simulink model "c00005M_harness"  (R2018a)
settings: Solver=FixedStepAuto  StartTime=0.0  StopTime=300  FixedStep=0.1  RelTol=1e-3
undefined symbols (not defined in the file): A1, hmax, PriorityTank, R1, R2, sigbuilder_block, TempThreshold
(part 44 of 50)

== system c00005M_harness/M203/Tank1/Control/Maintenance ==
  Type : Inport
  StartMaintenance : Inport  Port=2
  LiquidLevel : Inport  Port=3
  Chart : Stateflow chart  TreatAsAtomicUnit=on
  LiquidIn : Outport
  LiquidOut : Outport  Port=2
  wires:
  StartMaintenance/1 -> Chart/2(StartMaintenance)
  Type/1 -> Chart/1(Type)
  LiquidLevel/1 -> Chart/3(LiquidLevel)
  Chart/1(LiquidIn) -> LiquidIn/1
  Chart/2(LiquidOut) -> LiquidOut/1

== system c00005M_harness/M203/Tank1/Control/ManualControlLiquidInOut ==
  Fill : Inport
  Empty : Inport  Port=2
  LiquidLevel : Inport  Port=3
  Constant : Constant  Value=hmax*0.9
  Constant1 : Constant  Value=0.001
  Logical Operator{,1..2,4} (4 alike) : Logic  AllPortsSameDT=off  OutDataTypeStr=boolean
  Logical Operator3 : Logic  Operator=NOT  AllPortsSameDT=off  OutDataTypeStr=boolean
  Logical Operator5 : Logic  Operator=NOT  AllPortsSameDT=off  OutDataTypeStr=boolean
  Relational Operator1 : RelationalOperator  Operator=<  OutDataTypeStr=boolean  RndMeth=Simplest
  Relational Operator2 : RelationalOperator  Operator=<  OutDataTypeStr=boolean  RndMeth=Simplest
  LiquidIn : Outport
  LiquidOut : Outport  Port=2
  wires:
  Empty/1 -> Logical Operator1/2
  Constant/1 -> Relational Operator1/2
  Relational Operator1/1 -> Logical Operator/2
  Fill/1 -> Logical Operator/1
  Logical Operator/1 -> Logical Operator5/1, Logical Operator2/1
  Relational Operator2/1 -> Logical Operator1/1
  Logical Operator1/1 -> Logical Operator3/1, Logical Operator4/2
  Constant1/1 -> Relational Operator2/1
  LiquidLevel/1 -> Relational Operator2/2, Relational Operator1/1
  Logical Operator3/1 -> Logical Operator2/2
  Logical Operator2/1 -> LiquidIn/1
  Logical Operator5/1 -> Logical Operator4/1
  Logical Operator4/1 -> LiquidOut/1

== system c00005M_harness/M203/Tank3/Control/Maintenance ==
  Type : Inport
  StartMaintenance : Inport  Port=2
  LiquidLevel : Inport  Port=3
  Chart : Stateflow chart  TreatAsAtomicUnit=on
  LiquidIn : Outport
  LiquidOut : Outport  Port=2
  wires:
  StartMaintenance/1 -> Chart/2(StartMaintenance)
  Type/1 -> Chart/1(Type)
  LiquidLevel/1 -> Chart/3(LiquidLevel)
  Chart/1(LiquidIn) -> LiquidIn/1
  Chart/2(LiquidOut) -> LiquidOut/1

== system c00005M_harness/M203/Tank3/Control/ManualControlLiquidInOut ==
  Fill : Inport
  Empty : Inport  Port=2
  LiquidLevel : Inport  Port=3
  Constant : Constant  Value=hmax*0.9
  Constant1 : Constant  Value=0.001
  Logical Operator : Logic  AllPortsSameDT=off  OutDataTypeStr=boolean
  Logical Operator1 : Logic  Operator=OR  AllPortsSameDT=off  OutDataTypeStr=boolean
  Logical Operator2 : Logic  AllPortsSameDT=off  OutDataTypeStr=boolean
  Logical Operator3 : Logic  Operator=NOT  AllPortsSameDT=off  OutDataTypeStr=boolean
  Logical Operator4 : Logic  AllPortsSameDT=off  OutDataTypeStr=boolean
  Logical Operator5 : Logic  Operator=NOT  AllPortsSameDT=off  OutDataTypeStr=boolean
  Relational Operator1 : RelationalOperator  Operator=<  OutDataTypeStr=boolean  RndMeth=Simplest
  Relational Operator2 : RelationalOperator  Operator=<  OutDataTypeStr=boolean  RndMeth=Simplest
  LiquidIn : Outport
  LiquidOut : Outport  Port=2
  wires:
  Empty/1 -> Logical Operator1/2
  Constant/1 -> Relational Operator1/2
  Relational Operator1/1 -> Logical Operator/2
  Fill/1 -> Logical Operator/1
  Logical Operator/1 -> Logical Operator5/1, Logical Operator2/1
  Relational Operator2/1 -> Logical Operator1/1
  Logical Operator1/1 -> Logical Operator3/1, Logical Operator4/2
  Constant1/1 -> Relational Operator2/1
  LiquidLevel/1 -> Relational Operator2/2, Relational Operator1/1
  Logical Operator3/1 -> Logical Operator2/2
  Logical Operator2/1 -> LiquidIn/1
  Logical Operator5/1 -> Logical Operator4/1
  Logical Operator4/1 -> LiquidOut/1

== system c00005M_harness/M204/Tank1/Control/Maintenance ==
  Type : Inport
  StartMaintenance : Inport  Port=2
  LiquidLevel : Inport  Port=3
  Chart : Stateflow chart  TreatAsAtomicUnit=on
  LiquidIn : Outport
  LiquidOut : Outport  Port=2
  wires:
  StartMaintenance/1 -> Chart/2(StartMaintenance)
  Type/1 -> Chart/1(Type)
  LiquidLevel/1 -> Chart/3(LiquidLevel)
  Chart/1(LiquidIn) -> LiquidIn/1
  Chart/2(LiquidOut) -> LiquidOut/1

== system c00005M_harness/M204/Tank1/Control/ManualControlLiquidInOut ==
  Fill : Inport
  Empty : Inport  Port=2
  LiquidLevel : Inport  Port=3
  Constant : Constant  Value=hmax*0.9
  Constant1 : Constant  Value=0.001
  Logical Operator{,1..2,4} (4 alike) : Logic  AllPortsSameDT=off  OutDataTypeStr=boolean
  Logical Operator3 : Logic  Operator=NOT  AllPortsSameDT=off  OutDataTypeStr=boolean
  Logical Operator5 : Logic  Operator=NOT  AllPortsSameDT=off  OutDataTypeStr=boolean
  Relational Operator1 : RelationalOperator  Operator=<  OutDataTypeStr=boolean  RndMeth=Simplest
  Relational Operator2 : RelationalOperator  Operator=<  OutDataTypeStr=boolean  RndMeth=Simplest
  LiquidIn : Outport
  LiquidOut : Outport  Port=2
  wires:
  Empty/1 -> Logical Operator1/2
  Constant/1 -> Relational Operator1/2
  Relational Operator1/1 -> Logical Operator/2
  Fill/1 -> Logical Operator/1
  Logical Operator/1 -> Logical Operator5/1, Logical Operator2/1
  Relational Operator2/1 -> Logical Operator1/1
  Logical Operator1/1 -> Logical Operator3/1, Logical Operator4/2
  Constant1/1 -> Relational Operator2/1
  LiquidLevel/1 -> Relational Operator2/2, Relational Operator1/1
  Logical Operator3/1 -> Logical Operator2/2
  Logical Operator2/1 -> LiquidIn/1
  Logical Operator5/1 -> Logical Operator4/1
  Logical Operator4/1 -> LiquidOut/1

== system c00005M_harness/M204/Tank3/Control/Maintenance ==
  Type : Inport
  StartMaintenance : Inport  Port=2
  LiquidLevel : Inport  Port=3
  Chart : Stateflow chart  TreatAsAtomicUnit=on
  LiquidIn : Outport
  LiquidOut : Outport  Port=2
  wires:
  StartMaintenance/1 -> Chart/2(StartMaintenance)
  Type/1 -> Chart/1(Type)
  LiquidLevel/1 -> Chart/3(LiquidLevel)
  Chart/1(LiquidIn) -> LiquidIn/1
  Chart/2(LiquidOut) -> LiquidOut/1

== system c00005M_harness/M204/Tank3/Control/ManualControlLiquidInOut ==
  Fill : Inport
  Empty : Inport  Port=2
  LiquidLevel : Inport  Port=3
  Constant : Constant  Value=hmax*0.9
  Constant1 : Constant  Value=0.001
  Logical Operator : Logic  AllPortsSameDT=off  OutDataTypeStr=boolean
  Logical Operator1 : Logic  AllPortsSameDT=off  OutDataTypeStr=boolean
  Logical Operator2 : Logic  Operator=OR  AllPortsSameDT=off  OutDataTypeStr=boolean
  Logical Operator3 : Logic  Operator=NOT  AllPortsSameDT=off  OutDataTypeStr=boolean
  Logical Operator4 : Logic  AllPortsSameDT=off  OutDataTypeStr=boolean
  Logical Operator5 : Logic  Operator=NOT  AllPortsSameDT=off  OutDataTypeStr=boolean
  Relational Operator1 : RelationalOperator  Operator=<  OutDataTypeStr=boolean  RndMeth=Simplest
  Relational Operator2 : RelationalOperator  Operator=<  OutDataTypeStr=boolean  RndMeth=Simplest
  LiquidIn : Outport
  LiquidOut : Outport  Port=2
  wires:
  Empty/1 -> Logical Operator1/2
  Constant/1 -> Relational Operator1/2
  Relational Operator1/1 -> Logical Operator/2
  Fill/1 -> Logical Operator/1
  Logical Operator/1 -> Logical Operator5/1, Logical Operator2/1
  Relational Operator2/1 -> Logical Operator1/1
  Logical Operator1/1 -> Logical Operator3/1, Logical Operator4/2
  Constant1/1 -> Relational Operator2/1
  LiquidLevel/1 -> Relational Operator2/2, Relational Operator1/1
  Logical Operator3/1 -> Logical Operator2/2
  Logical Operator2/1 -> LiquidIn/1
  Logical Operator5/1 -> Logical Operator4/1
  Logical Operator4/1 -> LiquidOut/1

== system c00005M_harness/M205/Tank1/Control/Maintenance ==
  Type : Inport
  StartMaintenance : Inport  Port=2
  LiquidLevel : Inport  Port=3
  Chart : Stateflow chart  TreatAsAtomicUnit=on
  LiquidIn : Outport
  LiquidOut : Outport  Port=2
  wires:
  StartMaintenance/1 -> Chart/2(StartMaintenance)
  Type/1 -> Chart/1(Type)
  LiquidLevel/1 -> Chart/3(LiquidLevel)
  Chart/1(LiquidIn) -> LiquidIn/1
  Chart/2(LiquidOut) -> LiquidOut/1

== system c00005M_harness/M205/Tank1/Control/ManualControlLiquidInOut ==
  Fill : Inport
  Empty : Inport  Port=2
  LiquidLevel : Inport  Port=3
  Constant : Constant  Value=hmax*0.9
  Constant1 : Constant  Value=0.001
  Logical Operator{,1..2,4} (4 alike) : Logic  AllPortsSameDT=off  OutDataTypeStr=boolean
  Logical Operator3 : Logic  Operator=NOT  AllPortsSameDT=off  OutDataTypeStr=boolean
  Logical Operator5 : Logic  Operator=NOT  AllPortsSameDT=off  OutDataTypeStr=boolean
  Relational Operator1 : RelationalOperator  Operator=<  OutDataTypeStr=boolean  RndMeth=Simplest
  Relational Operator2 : RelationalOperator  Operator=<  OutDataTypeStr=boolean  RndMeth=Simplest
  LiquidIn : Outport
  LiquidOut : Outport  Port=2
  wires:
  Empty/1 -> Logical Operator1/2
  Constant/1 -> Relational Operator1/2
  Relational Operator1/1 -> Logical Operator/2
  Fill/1 -> Logical Operator/1
  Logical Operator/1 -> Logical Operator5/1, Logical Operator2/1
  Relational Operator2/1 -> Logical Operator1/1
  Logical Operator1/1 -> Logical Operator3/1, Logical Operator4/2
  Constant1/1 -> Relational Operator2/1
  LiquidLevel/1 -> Relational Operator2/2, Relational Operator1/1
  Logical Operator3/1 -> Logical Operator2/2
  Logical Operator2/1 -> LiquidIn/1
  Logical Operator5/1 -> Logical Operator4/1
  Logical Operator4/1 -> LiquidOut/1

== system c00005M_harness/M205/Tank3/Control/Maintenance ==
  Type : Inport
  StartMaintenance : Inport  Port=2
  LiquidLevel : Inport  Port=3
  Chart : Stateflow chart  TreatAsAtomicUnit=on
  LiquidIn : Outport
  LiquidOut : Outport  Port=2
  wires:
  StartMaintenance/1 -> Chart/2(StartMaintenance)
  Type/1 -> Chart/1(Type)
  LiquidLevel/1 -> Chart/3(LiquidLevel)
  Chart/1(LiquidIn) -> LiquidIn/1
  Chart/2(LiquidOut) -> LiquidOut/1

== system c00005M_harness/M205/Tank3/Control/ManualControlLiquidInOut ==
  Fill : Inport
  Empty : Inport  Port=2
  LiquidLevel : Inport  Port=3
  Constant : Constant  Value=hmax*0.9
  Constant1 : Constant  Value=0.001
  Logical Operator{,1..2,4} (4 alike) : Logic  AllPortsSameDT=off  OutDataTypeStr=boolean
  Logical Operator5 : Logic  Operator=NOT  AllPortsSameDT=off  OutDataTypeStr=boolean
  Relational Operator1 : RelationalOperator  Operator=<  OutDataTypeStr=boolean  RndMeth=Simplest
  Relational Operator2 : RelationalOperator  Operator=<  OutDataTypeStr=boolean  RndMeth=Simplest
  LiquidIn : Outport
  LiquidOut : Outport  Port=2
  wires:
  Empty/1 -> Logical Operator1/2
  Constant/1 -> Relational Operator1/2
  Relational Operator1/1 -> Logical Operator/2
  Fill/1 -> Logical Operator/1
  Logical Operator/1 -> Logical Operator5/1, Logical Operator2/1
  Relational Operator2/1 -> Logical Operator1/1
  Constant1/1 -> Relational Operator2/1
  LiquidLevel/1 -> Relational Operator2/2, Relational Operator1/1
  Logical Operator1/1 -> Logical Operator2/2, Logical Operator4/2
  Logical Operator2/1 -> LiquidIn/1
  Logical Operator5/1 -> Logical Operator4/1
  Logical Operator4/1 -> LiquidOut/1

== system c00005M_harness/M206/Tank1/Control/Maintenance ==
  Type : Inport
  StartMaintenance : Inport  Port=2
  LiquidLevel : Inport  Port=3
  Chart : Stateflow chart  TreatAsAtomicUnit=on
  LiquidIn : Outport
  LiquidOut : Outport  Port=2
  wires:
  StartMaintenance/1 -> Chart/2(StartMaintenance)
  Type/1 -> Chart/1(Type)
  LiquidLevel/1 -> Chart/3(LiquidLevel)
  Chart/1(LiquidIn) -> LiquidIn/1
  Chart/2(LiquidOut) -> LiquidOut/1

== system c00005M_harness/M206/Tank1/Control/ManualControlLiquidInOut ==
  Fill : Inport
  Empty : Inport  Port=2
  LiquidLevel : Inport  Port=3
  Constant : Constant  Value=hmax*0.9
  Constant1 : Constant  Value=0.001
  Logical Operator{,1..2,4} (4 alike) : Logic  AllPortsSameDT=off  OutDataTypeStr=boolean
  Logical Operator3 : Logic  Operator=NOT  AllPortsSameDT=off  OutDataTypeStr=boolean
  Logical Operator5 : Logic  Operator=NOT  AllPortsSameDT=off  OutDataTypeStr=boolean
  Relational Operator1 : RelationalOperator  Operator=<  OutDataTypeStr=boolean  RndMeth=Simplest
  Relational Operator2 : RelationalOperator  Operator=<  OutDataTypeStr=boolean  RndMeth=Simplest
  LiquidIn : Outport
  LiquidOut : Outport  Port=2
  wires:
  Empty/1 -> Logical Operator1/2
  Constant/1 -> Relational Operator1/2
  Relational Operator1/1 -> Logical Operator/2
  Fill/1 -> Logical Operator/1
  Logical Operator/1 -> Logical Operator5/1, Logical Operator2/1
  Relational Operator2/1 -> Logical Operator1/1
  Logical Operator1/1 -> Logical Operator3/1, Logical Operator4/2
  Constant1/1 -> Relational Operator2/1
  LiquidLevel/1 -> Relational Operator2/2, Relational Operator1/1
  Logical Operator3/1 -> Logical Operator2/2
  Logical Operator2/1 -> LiquidIn/1
  Logical Operator5/1 -> Logical Operator4/1
  Logical Operator4/1 -> LiquidOut/1

== system c00005M_harness/M206/Tank3/Control/Maintenance ==
  Type : Inport
  StartMaintenance : Inport  Port=2
  LiquidLevel : Inport  Port=3
  Chart : Stateflow chart  TreatAsAtomicUnit=on
  LiquidIn : Outport
  LiquidOut : Outport  Port=2
  wires:
  StartMaintenance/1 -> Chart/2(StartMaintenance)
  Type/1 -> Chart/1(Type)
  LiquidLevel/1 -> Chart/3(LiquidLevel)
  Chart/1(LiquidIn) -> LiquidIn/1
  Chart/2(LiquidOut) -> LiquidOut/1

== system c00005M_harness/M206/Tank3/Control/ManualControlLiquidInOut ==
  Fill : Inport
  Empty : Inport  Port=2
  LiquidLevel : Inport  Port=3
  Constant : Constant  Value=hmax*0.9
  Constant1 : Constant  Value=0.001
  Logical Operator : Logic  AllPortsSameDT=off  OutDataTypeStr=boolean
  Logical Operator1 : Logic  AllPortsSameDT=off  OutDataTypeStr=boolean
  Logical Operator2 : Logic  AllPortsSameDT=off  OutDataTypeStr=boolean
  Logical Operator3 : Logic  Operator=NOT  AllPortsSameDT=off  OutDataTypeStr=boolean
  Logical Operator4 : Logic  Operator=OR  AllPortsSameDT=off  OutDataTypeStr=boolean
  Logical Operator5 : Logic  Operator=NOT  AllPortsSameDT=off  OutDataTypeStr=boolean
  Relational Operator1 : RelationalOperator  Operator=<  OutDataTypeStr=boolean  RndMeth=Simplest
  Relational Operator2 : RelationalOperator  Operator=<  OutDataTypeStr=boolean  RndMeth=Simplest
  LiquidIn : Outport
  LiquidOut : Outport  Port=2
  wires:
  Empty/1 -> Logical Operator1/2
  Constant/1 -> Relational Operator1/2
  Relational Operator1/1 -> Logical Operator/2
  Fill/1 -> Logical Operator/1
  Logical Operator/1 -> Logical Operator5/1, Logical Operator2/1
  Relational Operator2/1 -> Logical Operator1/1
  Logical Operator1/1 -> Logical Operator3/1, Logical Operator4/2
  Constant1/1 -> Relational Operator2/1
  LiquidLevel/1 -> Relational Operator2/2, Relational Operator1/1
  Logical Operator3/1 -> Logical Operator2/2
  Logical Operator2/1 -> LiquidIn/1
  Logical Operator5/1 -> Logical Operator4/1
  Logical Operator4/1 -> LiquidOut/1

== system c00005M_harness/M207/Tank1/Control/Maintenance ==
  Type : Inport
  StartMaintenance : Inport  Port=2
  LiquidLevel : Inport  Port=3
  Chart : Stateflow chart  TreatAsAtomicUnit=on
  LiquidIn : Outport
  LiquidOut : Outport  Port=2
  wires:
  StartMaintenance/1 -> Chart/2(StartMaintenance)
  Type/1 -> Chart/1(Type)
  LiquidLevel/1 -> Chart/3(LiquidLevel)
  Chart/1(LiquidIn) -> LiquidIn/1
  Chart/2(LiquidOut) -> LiquidOut/1

== system c00005M_harness/M207/Tank1/Control/ManualControlLiquidInOut ==
  Fill : Inport
  Empty : Inport  Port=2
  LiquidLevel : Inport  Port=3
  Constant : Constant  Value=hmax*0.9
  Constant1 : Constant  Value=0.001
  Logical Operator{,1..2,4} (4 alike) : Logic  AllPortsSameDT=off  OutDataTypeStr=boolean
  Logical Operator3 : Logic  Operator=NOT  AllPortsSameDT=off  OutDataTypeStr=boolean
  Logical Operator5 : Logic  Operator=NOT  AllPortsSameDT=off  OutDataTypeStr=boolean
  Relational Operator1 : RelationalOperator  Operator=<  OutDataTypeStr=boolean  RndMeth=Simplest
  Relational Operator2 : RelationalOperator  Operator=<  OutDataTypeStr=boolean  RndMeth=Simplest
  LiquidIn : Outport
  LiquidOut : Outport  Port=2
  wires:
  Empty/1 -> Logical Operator1/2
  Constant/1 -> Relational Operator1/2
  Relational Operator1/1 -> Logical Operator/2
  Fill/1 -> Logical Operator/1
  Logical Operator/1 -> Logical Operator5/1, Logical Operator2/1
  Relational Operator2/1 -> Logical Operator1/1
  Logical Operator1/1 -> Logical Operator3/1, Logical Operator4/2
  Constant1/1 -> Relational Operator2/1
  LiquidLevel/1 -> Relational Operator2/2, Relational Operator1/1
  Logical Operator3/1 -> Logical Operator2/2
  Logical Operator2/1 -> LiquidIn/1
  Logical Operator5/1 -> Logical Operator4/1
  Logical Operator4/1 -> LiquidOut/1

== system c00005M_harness/M207/Tank3/Control/Maintenance ==
  Type : Inport
  StartMaintenance : Inport  Port=2
  LiquidLevel : Inport  Port=3
  Chart : Stateflow chart  TreatAsAtomicUnit=on
  LiquidIn : Outport
  LiquidOut : Outport  Port=2
  wires:
  StartMaintenance/1 -> Chart/2(StartMaintenance)
  Type/1 -> Chart/1(Type)
  LiquidLevel/1 -> Chart/3(LiquidLevel)
  Chart/1(LiquidIn) -> LiquidIn/1
  Chart/2(LiquidOut) -> LiquidOut/1

== system c00005M_harness/M207/Tank3/Control/ManualControlLiquidInOut ==
  Fill : Inport
  Empty : Inport  Port=2
  LiquidLevel : Inport  Port=3
  Constant : Constant  Value=hmax*0.9
  Constant1 : Constant  Value=0.001
  Logical Operator{,1..2,4} (4 alike) : Logic  AllPortsSameDT=off  OutDataTypeStr=boolean
  Logical Operator3 : Logic  Operator=NOT  AllPortsSameDT=off  OutDataTypeStr=boolean
  Relational Operator1 : RelationalOperator  Operator=<  OutDataTypeStr=boolean  RndMeth=Simplest
  Relational Operator2 : RelationalOperator  Operator=<  OutDataTypeStr=boolean  RndMeth=Simplest
  LiquidIn : Outport
  LiquidOut : Outport  Port=2
  wires:
  Empty/1 -> Logical Operator1/2
  Constant/1 -> Relational Operator1/2
  Relational Operator1/1 -> Logical Operator/2
  Fill/1 -> Logical Operator/1
  Relational Operator2/1 -> Logical Operator1/1
  Logical Operator1/1 -> Logical Operator3/1, Logical Operator4/2
  Constant1/1 -> Relational Operator2/1
  LiquidLevel/1 -> Relational Operator2/2, Relational Operator1/1
  Logical Operator3/1 -> Logical Operator2/2
  Logical Operator2/1 -> LiquidIn/1
  Logical Operator/1 -> Logical Operator4/1, Logical Operator2/1
  Logical Operator4/1 -> LiquidOut/1

== system c00005M_harness/M208/Tank1/Control/Maintenance ==
  Type : Inport
  StartMaintenance : Inport  Port=2
  LiquidLevel : Inport  Port=3
  Chart : Stateflow chart  TreatAsAtomicUnit=on
  LiquidIn : Outport
  LiquidOut : Outport  Port=2
  wires:
  StartMaintenance/1 -> Chart/2(StartMaintenance)
  Type/1 -> Chart/1(Type)
  LiquidLevel/1 -> Chart/3(LiquidLevel)
  Chart/1(LiquidIn) -> LiquidIn/1
  Chart/2(LiquidOut) -> LiquidOut/1

== system c00005M_harness/M208/Tank1/Control/ManualControlLiquidInOut ==
  Fill : Inport
  Empty : Inport  Port=2
  LiquidLevel : Inport  Port=3
  Constant : Constant  Value=hmax*0.9
  Constant1 : Constant  Value=0.001
  Logical Operator{,1..2,4} (4 alike) : Logic  AllPortsSameDT=off  OutDataTypeStr=boolean
  Logical Operator3 : Logic  Operator=NOT  AllPortsSameDT=off  OutDataTypeStr=boolean
  Logical Operator5 : Logic  Operator=NOT  AllPortsSameDT=off  OutDataTypeStr=boolean
  Relational Operator1 : RelationalOperator  Operator=<  OutDataTypeStr=boolean  RndMeth=Simplest
  Relational Operator2 : RelationalOperator  Operator=<  OutDataTypeStr=boolean  RndMeth=Simplest
  LiquidIn : Outport
  LiquidOut : Outport  Port=2
  wires:
  Empty/1 -> Logical Operator1/2
  Constant/1 -> Relational Operator1/2
  Relational Operator1/1 -> Logical Operator/2
  Fill/1 -> Logical Operator/1
  Logical Operator/1 -> Logical Operator5/1, Logical Operator2/1
  Relational Operator2/1 -> Logical Operator1/1
  Logical Operator1/1 -> Logical Operator3/1, Logical Operator4/2
  Constant1/1 -> Relational Operator2/1
  LiquidLevel/1 -> Relational Operator2/2, Relational Operator1/1
  Logical Operator3/1 -> Logical Operator2/2
  Logical Operator2/1 -> LiquidIn/1
  Logical Operator5/1 -> Logical Operator4/1
  Logical Operator4/1 -> LiquidOut/1

== system c00005M_harness/M208/Tank3/Control/Maintenance ==
  Type : Inport
  StartMaintenance : Inport  Port=2
  LiquidLevel : Inport  Port=3
  Chart : Stateflow chart  TreatAsAtomicUnit=on
  LiquidIn : Outport
  LiquidOut : Outport  Port=2
  wires:
  StartMaintenance/1 -> Chart/2(StartMaintenance)
  Type/1 -> Chart/1(Type)
  LiquidLevel/1 -> Chart/3(LiquidLevel)
  Chart/1(LiquidIn) -> LiquidIn/1
  Chart/2(LiquidOut) -> LiquidOut/1

== system c00005M_harness/M208/Tank3/Control/ManualControlLiquidInOut ==
  Fill : Inport
  Empty : Inport  Port=2
  LiquidLevel : Inport  Port=3
  Constant : Constant  Value=hmax*0.9
  Constant1 : Constant  Value=0.001
  Logical Operator{,1..2,4} (4 alike) : Logic  AllPortsSameDT=off  OutDataTypeStr=boolean
  Logical Operator3 : Logic  Operator=NOT  AllPortsSameDT=off  OutDataTypeStr=boolean
  Logical Operator5 : Logic  Operator=NOT  AllPortsSameDT=off  OutDataTypeStr=boolean
  Relational Operator1 : RelationalOperator  Operator=>  OutDataTypeStr=boolean  RndMeth=Simplest
  Relational Operator2 : RelationalOperator  Operator=<  OutDataTypeStr=boolean  RndMeth=Simplest
  LiquidIn : Outport
  LiquidOut : Outport  Port=2
  wires:
  Empty/1 -> Logical Operator1/2
  Constant/1 -> Relational Operator1/2
  Relational Operator1/1 -> Logical Operator/2
  Fill/1 -> Logical Operator/1
  Logical Operator/1 -> Logical Operator5/1, Logical Operator2/1
  Relational Operator2/1 -> Logical Operator1/1
  Logical Operator1/1 -> Logical Operator3/1, Logical Operator4/2
  Constant1/1 -> Relational Operator2/1
  LiquidLevel/1 -> Relational Operator2/2, Relational Operator1/1
  Logical Operator3/1 -> Logical Operator2/2
  Logical Operator2/1 -> LiquidIn/1
  Logical Operator5/1 -> Logical Operator4/1
  Logical Operator4/1 -> LiquidOut/1

== system c00005M_harness/M209/Tank1/Control/Maintenance ==
  Type : Inport
  StartMaintenance : Inport  Port=2
  LiquidLevel : Inport  Port=3
  Chart : Stateflow chart  TreatAsAtomicUnit=on
  LiquidIn : Outport
  LiquidOut : Outport  Port=2
  wires:
  StartMaintenance/1 -> Chart/2(StartMaintenance)
  Type/1 -> Chart/1(Type)
  LiquidLevel/1 -> Chart/3(LiquidLevel)
  Chart/1(LiquidIn) -> LiquidIn/1
  Chart/2(LiquidOut) -> LiquidOut/1

== system c00005M_harness/M209/Tank1/Control/ManualControlLiquidInOut ==
  Fill : Inport
  Empty : Inport  Port=2
  LiquidLevel : Inport  Port=3
  Constant : Constant  Value=hmax*0.9
  Constant1 : Constant  Value=0.001
  Logical Operator{,1..2,4} (4 alike) : Logic  AllPortsSameDT=off  OutDataTypeStr=boolean
  Logical Operator3 : Logic  Operator=NOT  AllPortsSameDT=off  OutDataTypeStr=boolean
  Logical Operator5 : Logic  Operator=NOT  AllPortsSameDT=off  OutDataTypeStr=boolean
  Relational Operator1 : RelationalOperator  Operator=<  OutDataTypeStr=boolean  RndMeth=Simplest
  Relational Operator2 : RelationalOperator  Operator=<  OutDataTypeStr=boolean  RndMeth=Simplest
  LiquidIn : Outport
  LiquidOut : Outport  Port=2
  wires:
  Empty/1 -> Logical Operator1/2
  Constant/1 -> Relational Operator1/2
  Relational Operator1/1 -> Logical Operator/2
  Fill/1 -> Logical Operator/1
  Logical Operator/1 -> Logical Operator5/1, Logical Operator2/1
  Relational Operator2/1 -> Logical Operator1/1
  Logical Operator1/1 -> Logical Operator3/1, Logical Operator4/2
  Constant1/1 -> Relational Operator2/1
  LiquidLevel/1 -> Relational Operator2/2, Relational Operator1/1
  Logical Operator3/1 -> Logical Operator2/2
  Logical Operator2/1 -> LiquidIn/1
  Logical Operator5/1 -> Logical Operator4/1
  Logical Operator4/1 -> LiquidOut/1

== system c00005M_harness/M209/Tank3/Control/Maintenance ==
  Type : Inport
  StartMaintenance : Inport  Port=2
  LiquidLevel : Inport  Port=3
  Chart : Stateflow chart  TreatAsAtomicUnit=on
  LiquidIn : Outport
  LiquidOut : Outport  Port=2
  wires:
  StartMaintenance/1 -> Chart/2(StartMaintenance)
  Type/1 -> Chart/1(Type)
  LiquidLevel/1 -> Chart/3(LiquidLevel)
  Chart/1(LiquidIn) -> LiquidIn/1
  Chart/2(LiquidOut) -> LiquidOut/1

== system c00005M_harness/M209/Tank3/Control/ManualControlLiquidInOut ==
  Fill : Inport
  Empty : Inport  Port=2
  LiquidLevel : Inport  Port=3
  Constant : Constant  Value=hmax*0.9
  Constant1 : Constant  Value=0.001
  Logical Operator{,1..2,4} (4 alike) : Logic  AllPortsSameDT=off  OutDataTypeStr=boolean
  Logical Operator3 : Logic  Operator=NOT  AllPortsSameDT=off  OutDataTypeStr=boolean
  Logical Operator5 : Logic  Operator=NOT  AllPortsSameDT=off  OutDataTypeStr=boolean
  Relational Operator1 : RelationalOperator  Operator=<  OutDataTypeStr=boolean  RndMeth=Simplest
  Relational Operator2 : RelationalOperator  Operator=>  OutDataTypeStr=boolean  RndMeth=Simplest
  LiquidIn : Outport
  LiquidOut : Outport  Port=2
  wires:
  Empty/1 -> Logical Operator1/2
  Constant/1 -> Relational Operator1/2
  Relational Operator1/1 -> Logical Operator/2
  Fill/1 -> Logical Operator/1
  Logical Operator/1 -> Logical Operator5/1, Logical Operator2/1
  Relational Operator2/1 -> Logical Operator1/1
  Logical Operator1/1 -> Logical Operator3/1, Logical Operator4/2
  Constant1/1 -> Relational Operator2/1
  LiquidLevel/1 -> Relational Operator2/2, Relational Operator1/1
  Logical Operator3/1 -> Logical Operator2/2
  Logical Operator2/1 -> LiquidIn/1
  Logical Operator5/1 -> Logical Operator4/1
  Logical Operator4/1 -> LiquidOut/1

== system c00005M_harness/M221/Tank1/Control/Maintenance ==
  Type : Inport
  StartMaintenance : Inport  Port=2
  LiquidLevel : Inport  Port=3
  Chart : Stateflow chart  TreatAsAtomicUnit=on
  LiquidIn : Outport
  LiquidOut : Outport  Port=2
  wires:
  StartMaintenance/1 -> Chart/2(StartMaintenance)
  Type/1 -> Chart/1(Type)
  LiquidLevel/1 -> Chart/3(LiquidLevel)
  Chart/1(LiquidIn) -> LiquidIn/1
  Chart/2(LiquidOut) -> LiquidOut/1

== system c00005M_harness/M221/Tank1/Control/ManualControlLiquidInOut ==
  Fill : Inport
  Empty : Inport  Port=2
  LiquidLevel : Inport  Port=3
  Constant : Constant  Value=hmax*0.9
  Constant1 : Constant  Value=0.001
  Logical Operator{,1..2,4} (4 alike) : Logic  AllPortsSameDT=off  OutDataTypeStr=boolean
  Logical Operator3 : Logic  Operator=NOT  AllPortsSameDT=off  OutDataTypeStr=boolean
  Logical Operator5 : Logic  Operator=NOT  AllPortsSameDT=off  OutDataTypeStr=boolean
  Relational Operator1 : RelationalOperator  Operator=<  OutDataTypeStr=boolean  RndMeth=Simplest
  Relational Operator2 : RelationalOperator  Operator=<  OutDataTypeStr=boolean  RndMeth=Simplest
  LiquidIn : Outport
  LiquidOut : Outport  Port=2
  wires:
  Empty/1 -> Logical Operator1/2
  Constant/1 -> Relational Operator1/2
  Relational Operator1/1 -> Logical Operator/2
  Fill/1 -> Logical Operator/1
  Logical Operator/1 -> Logical Operator5/1, Logical Operator2/1
  Relational Operator2/1 -> Logical Operator1/1
  Logical Operator1/1 -> Logical Operator3/1, Logical Operator4/2
  Constant1/1 -> Relational Operator2/1
  LiquidLevel/1 -> Relational Operator2/2, Relational Operator1/1
  Logical Operator3/1 -> Logical Operator2/2
  Logical Operator2/1 -> LiquidIn/1
  Logical Operator5/1 -> Logical Operator4/1
  Logical Operator4/1 -> LiquidOut/1

== system c00005M_harness/M221/Tank3/Control/Maintenance ==
  Type : Inport
  StartMaintenance : Inport  Port=2
  LiquidLevel : Inport  Port=3
  Chart : Stateflow chart  TreatAsAtomicUnit=on
  LiquidIn : Outport
  LiquidOut : Outport  Port=2
  wires:
  StartMaintenance/1 -> Chart/2(StartMaintenance)
  Type/1 -> Chart/1(Type)
  LiquidLevel/1 -> Chart/3(LiquidLevel)
  Chart/1(LiquidIn) -> LiquidIn/1
  Chart/2(LiquidOut) -> LiquidOut/1

== system c00005M_harness/M221/Tank3/Control/ManualControlLiquidInOut ==
  Fill : Inport
  Empty : Inport  Port=2
  LiquidLevel : Inport  Port=3
  Constant : Constant  Value=hmax*0.9
  Constant1 : Constant  Value=0.001
  Logical Operator{,1..2,4} (4 alike) : Logic  AllPortsSameDT=off  OutDataTypeStr=boolean
  Logical Operator3 : Logic  Operator=NOT  AllPortsSameDT=off  OutDataTypeStr=boolean
  Logical Operator5 : Logic  Operator=NOT  AllPortsSameDT=off  OutDataTypeStr=boolean
  Relational Operator1 : RelationalOperator  Operator=<  OutDataTypeStr=boolean  RndMeth=Simplest
  Relational Operator2 : RelationalOperator  Operator=<  OutDataTypeStr=boolean  RndMeth=Simplest
  LiquidIn : Outport
  LiquidOut : Outport  Port=2
  wires:
  Empty/1 -> Logical Operator1/2
  Constant/1 -> Relational Operator1/2
  Relational Operator1/1 -> Logical Operator/2
  Fill/1 -> Logical Operator/1
  Logical Operator/1 -> Logical Operator5/1, Logical Operator2/1
  Relational Operator2/1 -> Logical Operator1/1
  Logical Operator1/1 -> Logical Operator3/1, Logical Operator4/2
  Constant1/1 -> Relational Operator2/1
  LiquidLevel/1 -> Relational Operator2/2, Relational Operator1/1
  Logical Operator3/1 -> Logical Operator2/2
  Logical Operator2/1 -> LiquidIn/1
  Logical Operator5/1 -> Logical Operator4/1
  Logical Operator4/1 -> LiquidOut/1

== system c00005M_harness/M222/Tank1/Control/Maintenance ==
  Type : Inport
  StartMaintenance : Inport  Port=2
  LiquidLevel : Inport  Port=3
  Chart : Stateflow chart  TreatAsAtomicUnit=on
  LiquidIn : Outport
  LiquidOut : Outport  Port=2
  wires:
  StartMaintenance/1 -> Chart/2(StartMaintenance)
  Type/1 -> Chart/1(Type)
  LiquidLevel/1 -> Chart/3(LiquidLevel)
  Chart/1(LiquidIn) -> LiquidIn/1
  Chart/2(LiquidOut) -> LiquidOut/1

== system c00005M_harness/M222/Tank1/Control/ManualControlLiquidInOut ==
  Fill : Inport
  Empty : Inport  Port=2
  LiquidLevel : Inport  Port=3
  Constant : Constant  Value=hmax*0.9
  Constant1 : Constant  Value=0.001
  Logical Operator{,1..2,4} (4 alike) : Logic  AllPortsSameDT=off  OutDataTypeStr=boolean
  Logical Operator3 : Logic  Operator=NOT  AllPortsSameDT=off  OutDataTypeStr=boolean
  Logical Operator5 : Logic  Operator=NOT  AllPortsSameDT=off  OutDataTypeStr=boolean
  Relational Operator1 : RelationalOperator  Operator=<  OutDataTypeStr=boolean  RndMeth=Simplest
  Relational Operator2 : RelationalOperator  Operator=<  OutDataTypeStr=boolean  RndMeth=Simplest
  LiquidIn : Outport
  LiquidOut : Outport  Port=2
  wires:
  Empty/1 -> Logical Operator1/2
  Constant/1 -> Relational Operator1/2
  Relational Operator1/1 -> Logical Operator/2
  Fill/1 -> Logical Operator/1
  Logical Operator/1 -> Logical Operator5/1, Logical Operator2/1
  Relational Operator2/1 -> Logical Operator1/1
  Logical Operator1/1 -> Logical Operator3/1, Logical Operator4/2
  Constant1/1 -> Relational Operator2/1
  LiquidLevel/1 -> Relational Operator2/2, Relational Operator1/1
  Logical Operator3/1 -> Logical Operator2/2
  Logical Operator2/1 -> LiquidIn/1
  Logical Operator5/1 -> Logical Operator4/1
  Logical Operator4/1 -> LiquidOut/1

== system c00005M_harness/M222/Tank3/Control/Maintenance ==
  Type : Inport
  StartMaintenance : Inport  Port=2
  LiquidLevel : Inport  Port=3
  Chart : Stateflow chart  TreatAsAtomicUnit=on
  LiquidIn : Outport
  LiquidOut : Outport  Port=2
  wires:
  StartMaintenance/1 -> Chart/2(StartMaintenance)
  Type/1 -> Chart/1(Type)
  LiquidLevel/1 -> Chart/3(LiquidLevel)
  Chart/1(LiquidIn) -> LiquidIn/1
  Chart/2(LiquidOut) -> LiquidOut/1

== system c00005M_harness/M222/Tank3/Control/ManualControlLiquidInOut ==
  Fill : Inport
  Empty : Inport  Port=2
  LiquidLevel : Inport  Port=3
  Constant : Constant  Value=hmax*0.9
  Constant1 : Constant  Value=0.001
  Logical Operator{,1..2,4} (4 alike) : Logic  AllPortsSameDT=off  OutDataTypeStr=boolean
  Logical Operator3 : Logic  Operator=NOT  AllPortsSameDT=off  OutDataTypeStr=boolean
  Logical Operator5 : Logic  Operator=NOT  AllPortsSameDT=off  OutDataTypeStr=boolean
  Relational Operator1 : RelationalOperator  Operator=<  OutDataTypeStr=boolean  RndMeth=Simplest
  Relational Operator2 : RelationalOperator  Operator=<  OutDataTypeStr=boolean  RndMeth=Simplest
  LiquidIn : Outport
  LiquidOut : Outport  Port=2
  wires:
  Empty/1 -> Logical Operator1/2
  Constant/1 -> Relational Operator1/2
  Relational Operator1/1 -> Logical Operator/2
  Fill/1 -> Logical Operator/1
  Logical Operator/1 -> Logical Operator5/1, Logical Operator2/1
  Relational Operator2/1 -> Logical Operator1/1
  Logical Operator1/1 -> Logical Operator3/1, Logical Operator4/2
  Constant1/1 -> Relational Operator2/1
  LiquidLevel/1 -> Relational Operator2/2, Relational Operator1/1
  Logical Operator3/1 -> Logical Operator2/2
  Logical Operator2/1 -> LiquidIn/1
  Logical Operator5/1 -> Logical Operator4/1
  Logical Operator4/1 -> LiquidOut/1

== system c00005M_harness/M223/Tank1/Control/Maintenance ==
  Type : Inport
  StartMaintenance : Inport  Port=2
  LiquidLevel : Inport  Port=3
  Chart : Stateflow chart  TreatAsAtomicUnit=on
  LiquidIn : Outport
  LiquidOut : Outport  Port=2
  wires:
  StartMaintenance/1 -> Chart/2(StartMaintenance)
  Type/1 -> Chart/1(Type)
  LiquidLevel/1 -> Chart/3(LiquidLevel)
  Chart/1(LiquidIn) -> LiquidIn/1
  Chart/2(LiquidOut) -> LiquidOut/1

== system c00005M_harness/M223/Tank1/Control/ManualControlLiquidInOut ==
  Fill : Inport
  Empty : Inport  Port=2
  LiquidLevel : Inport  Port=3
  Constant : Constant  Value=hmax*0.9
  Constant1 : Constant  Value=0.001
  Logical Operator{,1..2,4} (4 alike) : Logic  AllPortsSameDT=off  OutDataTypeStr=boolean
  Logical Operator3 : Logic  Operator=NOT  AllPortsSameDT=off  OutDataTypeStr=boolean
  Logical Operator5 : Logic  Operator=NOT  AllPortsSameDT=off  OutDataTypeStr=boolean
  Relational Operator1 : RelationalOperator  Operator=<  OutDataTypeStr=boolean  RndMeth=Simplest
  Relational Operator2 : RelationalOperator  Operator=<  OutDataTypeStr=boolean  RndMeth=Simplest
  LiquidIn : Outport
  LiquidOut : Outport  Port=2
  wires:
  Empty/1 -> Logical Operator1/2
  Constant/1 -> Relational Operator1/2
  Relational Operator1/1 -> Logical Operator/2
  Fill/1 -> Logical Operator/1
  Logical Operator/1 -> Logical Operator5/1, Logical Operator2/1
  Relational Operator2/1 -> Logical Operator1/1
  Logical Operator1/1 -> Logical Operator3/1, Logical Operator4/2
  Constant1/1 -> Relational Operator2/1
  LiquidLevel/1 -> Relational Operator2/2, Relational Operator1/1
  Logical Operator3/1 -> Logical Operator2/2
  Logical Operator2/1 -> LiquidIn/1
  Logical Operator5/1 -> Logical Operator4/1
  Logical Operator4/1 -> LiquidOut/1

== system c00005M_harness/M223/Tank3/Control/Maintenance ==
  Type : Inport
  StartMaintenance : Inport  Port=2
  LiquidLevel : Inport  Port=3
  Chart : Stateflow chart  TreatAsAtomicUnit=on
  LiquidIn : Outport
  LiquidOut : Outport  Port=2
  wires:
  StartMaintenance/1 -> Chart/2(StartMaintenance)
  Type/1 -> Chart/1(Type)
  LiquidLevel/1 -> Chart/3(LiquidLevel)
  Chart/1(LiquidIn) -> LiquidIn/1
  Chart/2(LiquidOut) -> LiquidOut/1

== system c00005M_harness/M223/Tank3/Control/ManualControlLiquidInOut ==
  Fill : Inport
  Empty : Inport  Port=2
  LiquidLevel : Inport  Port=3
  Constant : Constant  Value=hmax*0.9
  Constant1 : Constant  Value=0.001
  Logical Operator{,1..2,4} (4 alike) : Logic  AllPortsSameDT=off  OutDataTypeStr=boolean
  Logical Operator3 : Logic  Operator=NOT  AllPortsSameDT=off  OutDataTypeStr=boolean
  Logical Operator5 : Logic  Operator=NOT  AllPortsSameDT=off  OutDataTypeStr=boolean
  Relational Operator1 : RelationalOperator  Operator=<  OutDataTypeStr=boolean  RndMeth=Simplest
  Relational Operator2 : RelationalOperator  Operator=<  OutDataTypeStr=boolean  RndMeth=Simplest
  LiquidIn : Outport
  LiquidOut : Outport  Port=2
  wires:
  Empty/1 -> Logical Operator1/2
  Constant/1 -> Relational Operator1/2
  Relational Operator1/1 -> Logical Operator/2
  Fill/1 -> Logical Operator/1
  Logical Operator/1 -> Logical Operator5/1, Logical Operator2/1
  Relational Operator2/1 -> Logical Operator1/1
  Logical Operator1/1 -> Logical Operator3/1, Logical Operator4/2
  Constant1/1 -> Relational Operator2/1
  LiquidLevel/1 -> Relational Operator2/2, Relational Operator1/1
  Logical Operator3/1 -> Logical Operator2/2
  Logical Operator2/1 -> LiquidIn/1
  Logical Operator5/1 -> Logical Operator4/1
  Logical Operator4/1 -> LiquidOut/1

== system c00005M_harness/M224/Tank1/Control/Maintenance ==
  Type : Inport
  StartMaintenance : Inport  Port=2
  LiquidLevel : Inport  Port=3
  Chart : Stateflow chart  TreatAsAtomicUnit=on
  LiquidIn : Outport
  LiquidOut : Outport  Port=2
  wires:
  StartMaintenance/1 -> Chart/2(StartMaintenance)
  Type/1 -> Chart/1(Type)
  LiquidLevel/1 -> Chart/3(LiquidLevel)
  Chart/1(LiquidIn) -> LiquidIn/1
  Chart/2(LiquidOut) -> LiquidOut/1

== system c00005M_harness/M224/Tank1/Control/ManualControlLiquidInOut ==
  Fill : Inport
  Empty : Inport  Port=2
  LiquidLevel : Inport  Port=3
  Constant : Constant  Value=hmax*0.9
  Constant1 : Constant  Value=0.001
  Logical Operator{,1..2,4} (4 alike) : Logic  AllPortsSameDT=off  OutDataTypeStr=boolean
  Logical Operator3 : Logic  Operator=NOT  AllPortsSameDT=off  OutDataTypeStr=boolean
  Logical Operator5 : Logic  Operator=NOT  AllPortsSameDT=off  OutDataTypeStr=boolean
  Relational Operator1 : RelationalOperator  Operator=<  OutDataTypeStr=boolean  RndMeth=Simplest
  Relational Operator2 : RelationalOperator  Operator=<  OutDataTypeStr=boolean  RndMeth=Simplest
  LiquidIn : Outport
  LiquidOut : Outport  Port=2
  wires:
  Empty/1 -> Logical Operator1/2
  Constant/1 -> Relational Operator1/2
  Relational Operator1/1 -> Logical Operator/2
  Fill/1 -> Logical Operator/1
  Logical Operator/1 -> Logical Operator5/1, Logical Operator2/1
  Relational Operator2/1 -> Logical Operator1/1
  Logical Operator1/1 -> Logical Operator3/1, Logical Operator4/2
  Constant1/1 -> Relational Operator2/1
  LiquidLevel/1 -> Relational Operator2/2, Relational Operator1/1
  Logical Operator3/1 -> Logical Operator2/2
  Logical Operator2/1 -> LiquidIn/1
  Logical Operator5/1 -> Logical Operator4/1
  Logical Operator4/1 -> LiquidOut/1

== system c00005M_harness/M224/Tank3/Control/Maintenance ==
  Type : Inport
  StartMaintenance : Inport  Port=2
  LiquidLevel : Inport  Port=3
  Chart : Stateflow chart  TreatAsAtomicUnit=on
  LiquidIn : Outport
  LiquidOut : Outport  Port=2
  wires:
  StartMaintenance/1 -> Chart/2(StartMaintenance)
  Type/1 -> Chart/1(Type)
  LiquidLevel/1 -> Chart/3(LiquidLevel)
  Chart/1(LiquidIn) -> LiquidIn/1
  Chart/2(LiquidOut) -> LiquidOut/1

== system c00005M_harness/M224/Tank3/Control/ManualControlLiquidInOut ==
  Fill : Inport
  Empty : Inport  Port=2
  LiquidLevel : Inport  Port=3
  Constant : Constant  Value=hmax*0.9
  Constant1 : Constant  Value=0.001
  Logical Operator{,1..2,4} (4 alike) : Logic  AllPortsSameDT=off  OutDataTypeStr=boolean
  Logical Operator3 : Logic  Operator=NOT  AllPortsSameDT=off  OutDataTypeStr=boolean
  Logical Operator5 : Logic  Operator=NOT  AllPortsSameDT=off  OutDataTypeStr=boolean
  Relational Operator1 : RelationalOperator  Operator=<  OutDataTypeStr=boolean  RndMeth=Simplest
  Relational Operator2 : RelationalOperator  Operator=<  OutDataTypeStr=boolean  RndMeth=Simplest
  LiquidIn : Outport
  LiquidOut : Outport  Port=2
  wires:
  Empty/1 -> Logical Operator1/2
  Constant/1 -> Relational Operator1/2
  Relational Operator1/1 -> Logical Operator/2
  Fill/1 -> Logical Operator/1
  Logical Operator/1 -> Logical Operator5/1, Logical Operator2/1
  Relational Operator2/1 -> Logical Operator1/1
  Logical Operator1/1 -> Logical Operator3/1, Logical Operator4/2
  Constant1/1 -> Relational Operator2/1
  LiquidLevel/1 -> Relational Operator2/2, Relational Operator1/1
  Logical Operator3/1 -> Logical Operator2/2
  Logical Operator2/1 -> LiquidIn/1
  Logical Operator5/1 -> Logical Operator4/1
  Logical Operator4/1 -> LiquidOut/1

== system c00005M_harness/M225/Tank1/Control/Maintenance ==
  Type : Inport
  StartMaintenance : Inport  Port=2
  LiquidLevel : Inport  Port=3
  Chart : Stateflow chart  TreatAsAtomicUnit=on
  LiquidIn : Outport
  LiquidOut : Outport  Port=2
  wires:
  StartMaintenance/1 -> Chart/2(StartMaintenance)
  Type/1 -> Chart/1(Type)
  LiquidLevel/1 -> Chart/3(LiquidLevel)
  Chart/1(LiquidIn) -> LiquidIn/1
  Chart/2(LiquidOut) -> LiquidOut/1

== system c00005M_harness/M225/Tank1/Control/ManualControlLiquidInOut ==
  Fill : Inport
  Empty : Inport  Port=2
  LiquidLevel : Inport  Port=3
  Constant : Constant  Value=hmax*0.9
  Constant1 : Constant  Value=0.001
  Logical Operator{,1..2,4} (4 alike) : Logic  AllPortsSameDT=off  OutDataTypeStr=boolean
  Logical Operator3 : Logic  Operator=NOT  AllPortsSameDT=off  OutDataTypeStr=boolean
  Logical Operator5 : Logic  Operator=NOT  AllPortsSameDT=off  OutDataTypeStr=boolean
  Relational Operator1 : RelationalOperator  Operator=<  OutDataTypeStr=boolean  RndMeth=Simplest
  Relational Operator2 : RelationalOperator  Operator=<  OutDataTypeStr=boolean  RndMeth=Simplest
  LiquidIn : Outport
  LiquidOut : Outport  Port=2
  wires:
  Empty/1 -> Logical Operator1/2
  Constant/1 -> Relational Operator1/2
  Relational Operator1/1 -> Logical Operator/2
  Fill/1 -> Logical Operator/1
  Logical Operator/1 -> Logical Operator5/1, Logical Operator2/1
  Relational Operator2/1 -> Logical Operator1/1
  Logical Operator1/1 -> Logical Operator3/1, Logical Operator4/2
  Constant1/1 -> Relational Operator2/1
  LiquidLevel/1 -> Relational Operator2/2, Relational Operator1/1
  Logical Operator3/1 -> Logical Operator2/2
  Logical Operator2/1 -> LiquidIn/1
  Logical Operator5/1 -> Logical Operator4/1
  Logical Operator4/1 -> LiquidOut/1

== system c00005M_harness/M225/Tank3/Control/Maintenance ==
  Type : Inport
  StartMaintenance : Inport  Port=2
  LiquidLevel : Inport  Port=3
  Chart : Stateflow chart  TreatAsAtomicUnit=on
  LiquidIn : Outport
  LiquidOut : Outport  Port=2
  wires:
  StartMaintenance/1 -> Chart/2(StartMaintenance)
  Type/1 -> Chart/1(Type)
  LiquidLevel/1 -> Chart/3(LiquidLevel)
  Chart/1(LiquidIn) -> LiquidIn/1
  Chart/2(LiquidOut) -> LiquidOut/1

== system c00005M_harness/M225/Tank3/Control/ManualControlLiquidInOut ==
  Fill : Inport
  Empty : Inport  Port=2
  LiquidLevel : Inport  Port=3
  Constant : Constant  Value=hmax*0.9
  Constant1 : Constant  Value=0.001
  Logical Operator{,1..2,4} (4 alike) : Logic  AllPortsSameDT=off  OutDataTypeStr=boolean
  Logical Operator3 : Logic  Operator=NOT  AllPortsSameDT=off  OutDataTypeStr=boolean
  Logical Operator5 : Logic  Operator=NOT  AllPortsSameDT=off  OutDataTypeStr=boolean
  Relational Operator1 : RelationalOperator  Operator=<  OutDataTypeStr=boolean  RndMeth=Simplest
  Relational Operator2 : RelationalOperator  Operator=<  OutDataTypeStr=boolean  RndMeth=Simplest
  LiquidIn : Outport
  LiquidOut : Outport  Port=2
  wires:
  Empty/1 -> Logical Operator1/2
  Constant/1 -> Relational Operator1/2
  Relational Operator1/1 -> Logical Operator/2
  Fill/1 -> Logical Operator/1
  Logical Operator/1 -> Logical Operator5/1, Logical Operator2/1
  Relational Operator2/1 -> Logical Operator1/1
  Logical Operator1/1 -> Logical Operator3/1, Logical Operator4/2
  Constant1/1 -> Relational Operator2/1
  LiquidLevel/1 -> Relational Operator2/2, Relational Operator1/1
  Logical Operator3/1 -> Logical Operator2/2
  Logical Operator2/1 -> LiquidIn/1
  Logical Operator5/1 -> Logical Operator4/1
  Logical Operator4/1 -> LiquidOut/1

== system c00005M_harness/M226/Tank1/Control/Maintenance ==
  Type : Inport
  StartMaintenance : Inport  Port=2
  LiquidLevel : Inport  Port=3
  Chart : Stateflow chart  TreatAsAtomicUnit=on
  LiquidIn : Outport
  LiquidOut : Outport  Port=2
  wires:
  StartMaintenance/1 -> Chart/2(StartMaintenance)
  Type/1 -> Chart/1(Type)
  LiquidLevel/1 -> Chart/3(LiquidLevel)
  Chart/1(LiquidIn) -> LiquidIn/1
  Chart/2(LiquidOut) -> LiquidOut/1

== system c00005M_harness/M226/Tank1/Control/ManualControlLiquidInOut ==
  Fill : Inport
  Empty : Inport  Port=2
  LiquidLevel : Inport  Port=3
  Constant : Constant  Value=hmax*0.9
  Constant1 : Constant  Value=0.001
  Logical Operator{,1..2,4} (4 alike) : Logic  AllPortsSameDT=off  OutDataTypeStr=boolean
  Logical Operator3 : Logic  Operator=NOT  AllPortsSameDT=off  OutDataTypeStr=boolean
  Logical Operator5 : Logic  Operator=NOT  AllPortsSameDT=off  OutDataTypeStr=boolean
  Relational Operator1 : RelationalOperator  Operator=<  OutDataTypeStr=boolean  RndMeth=Simplest
  Relational Operator2 : RelationalOperator  Operator=<  OutDataTypeStr=boolean  RndMeth=Simplest
  LiquidIn : Outport
  LiquidOut : Outport  Port=2
  wires:
  Empty/1 -> Logical Operator1/2
  Constant/1 -> Relational Operator1/2
  Relational Operator1/1 -> Logical Operator/2
  Fill/1 -> Logical Operator/1
  Logical Operator/1 -> Logical Operator5/1, Logical Operator2/1
  Relational Operator2/1 -> Logical Operator1/1
  Logical Operator1/1 -> Logical Operator3/1, Logical Operator4/2
  Constant1/1 -> Relational Operator2/1
  LiquidLevel/1 -> Relational Operator2/2, Relational Operator1/1
  Logical Operator3/1 -> Logical Operator2/2
  Logical Operator2/1 -> LiquidIn/1
  Logical Operator5/1 -> Logical Operator4/1
  Logical Operator4/1 -> LiquidOut/1

== system c00005M_harness/M226/Tank3/Control/Maintenance ==
  Type : Inport
  StartMaintenance : Inport  Port=2
  LiquidLevel : Inport  Port=3
  Chart : Stateflow chart  TreatAsAtomicUnit=on
  LiquidIn : Outport
  LiquidOut : Outport  Port=2
  wires:
  StartMaintenance/1 -> Chart/2(StartMaintenance)
  Type/1 -> Chart/1(Type)
  LiquidLevel/1 -> Chart/3(LiquidLevel)
  Chart/1(LiquidIn) -> LiquidIn/1
  Chart/2(LiquidOut) -> LiquidOut/1

== system c00005M_harness/M226/Tank3/Control/ManualControlLiquidInOut ==
  Fill : Inport
  Empty : Inport  Port=2
  LiquidLevel : Inport  Port=3
  Constant : Constant  Value=hmax*0.9
  Constant1 : Constant  Value=0.001
  Logical Operator{,1..2,4} (4 alike) : Logic  AllPortsSameDT=off  OutDataTypeStr=boolean
  Logical Operator3 : Logic  Operator=NOT  AllPortsSameDT=off  OutDataTypeStr=boolean
  Logical Operator5 : Logic  Operator=NOT  AllPortsSameDT=off  OutDataTypeStr=boolean
  Relational Operator1 : RelationalOperator  Operator=<  OutDataTypeStr=boolean  RndMeth=Simplest
  Relational Operator2 : RelationalOperator  Operator=<  OutDataTypeStr=boolean  RndMeth=Simplest
  LiquidIn : Outport
  LiquidOut : Outport  Port=2
  wires:
  Empty/1 -> Logical Operator1/2
  Constant/1 -> Relational Operator1/2
  Relational Operator1/1 -> Logical Operator/2
  Fill/1 -> Logical Operator/1
  Logical Operator/1 -> Logical Operator5/1, Logical Operator2/1
  Relational Operator2/1 -> Logical Operator1/1
  Logical Operator1/1 -> Logical Operator3/1, Logical Operator4/2
  Constant1/1 -> Relational Operator2/1
  LiquidLevel/1 -> Relational Operator2/2, Relational Operator1/1
  Logical Operator3/1 -> Logical Operator2/2
  Logical Operator2/1 -> LiquidIn/1
  Logical Operator5/1 -> Logical Operator4/1
  Logical Operator4/1 -> LiquidOut/1

== system c00005M_harness/M227/Tank1/Control/Maintenance ==
  Type : Inport
  StartMaintenance : Inport  Port=2
  LiquidLevel : Inport  Port=3
  Chart : Stateflow chart  TreatAsAtomicUnit=on
  LiquidIn : Outport
  LiquidOut : Outport  Port=2
  wires:
  StartMaintenance/1 -> Chart/2(StartMaintenance)
  Type/1 -> Chart/1(Type)
  LiquidLevel/1 -> Chart/3(LiquidLevel)
  Chart/1(LiquidIn) -> LiquidIn/1
  Chart/2(LiquidOut) -> LiquidOut/1

== system c00005M_harness/M227/Tank1/Control/ManualControlLiquidInOut ==
  Fill : Inport
  Empty : Inport  Port=2
  LiquidLevel : Inport  Port=3
  Constant : Constant  Value=hmax*0.9
  Constant1 : Constant  Value=0.001
  Logical Operator{,1..2,4} (4 alike) : Logic  AllPortsSameDT=off  OutDataTypeStr=boolean
  Logical Operator3 : Logic  Operator=NOT  AllPortsSameDT=off  OutDataTypeStr=boolean
  Logical Operator5 : Logic  Operator=NOT  AllPortsSameDT=off  OutDataTypeStr=boolean
  Relational Operator1 : RelationalOperator  Operator=<  OutDataTypeStr=boolean  RndMeth=Simplest
  Relational Operator2 : RelationalOperator  Operator=<  OutDataTypeStr=boolean  RndMeth=Simplest
  LiquidIn : Outport
  LiquidOut : Outport  Port=2
  wires:
  Empty/1 -> Logical Operator1/2
  Constant/1 -> Relational Operator1/2
  Relational Operator1/1 -> Logical Operator/2
  Fill/1 -> Logical Operator/1
  Logical Operator/1 -> Logical Operator5/1, Logical Operator2/1
  Relational Operator2/1 -> Logical Operator1/1
  Logical Operator1/1 -> Logical Operator3/1, Logical Operator4/2
  Constant1/1 -> Relational Operator2/1
  LiquidLevel/1 -> Relational Operator2/2, Relational Operator1/1
  Logical Operator3/1 -> Logical Operator2/2
  Logical Operator2/1 -> LiquidIn/1
  Logical Operator5/1 -> Logical Operator4/1
  Logical Operator4/1 -> LiquidOut/1

== system c00005M_harness/M227/Tank3/Control/Maintenance ==
  Type : Inport
  StartMaintenance : Inport  Port=2
  LiquidLevel : Inport  Port=3
  Chart : Stateflow chart  TreatAsAtomicUnit=on
  LiquidIn : Outport
  LiquidOut : Outport  Port=2
  wires:
  StartMaintenance/1 -> Chart/2(StartMaintenance)
  Type/1 -> Chart/1(Type)
  LiquidLevel/1 -> Chart/3(LiquidLevel)
  Chart/1(LiquidIn) -> LiquidIn/1
  Chart/2(LiquidOut) -> LiquidOut/1
